simulink model "main_servo_laser"  (R2019b)
settings: Solver=VariableStepAuto  StartTime=0.0  StopTime=60  RelTol=1e-3
undefined symbols (not defined in the file): __PRM__SERIALIZED__DATA__, SubsystemReferenceBlock
settings Model: Creator=toons  LastModifiedBy=toons

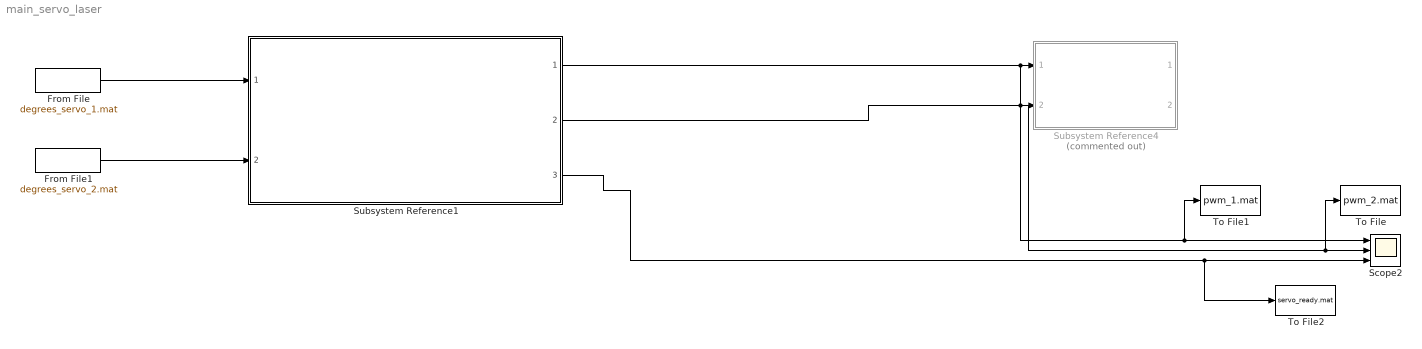
== system main_servo_laser ==
  From File : FromFile  FileName=degrees_servo_1.mat
  From File1 : FromFile  FileName=degrees_servo_2.mat
  Scope2 : Scope  NumInputPorts=3
  Subsystem Reference1 : Subsystem  BlockKeywords=__PRM__SERIALIZED__DATA__:SubsystemReferenceBlock  ReferencedSubsystem=MicroControllerPWM
  Subsystem Reference4 : Subsystem  Commented=on  BlockKeywords=__PRM__SERIALIZED__DATA__:SubsystemReferenceBlock  ReferencedSubsystem=ServoSimulation
  To File : ToFile  Filename=pwm_2.mat  SaveFormat=Timeseries
  To File1 : ToFile  Filename=pwm_1.mat  SaveFormat=Timeseries
  To File2 : ToFile  Filename=servo_ready.mat  SaveFormat=Timeseries
  wires:
  Subsystem Reference1/3 -> To File2/1, Scope2/3
  Subsystem Reference1/1 -> To File1/1, Scope2/1, Subsystem Reference4/1
  From File/1 -> Subsystem Reference1/1
  From File1/1 -> Subsystem Reference1/2
  Subsystem Reference1/2 -> To File/1, Scope2/2, Subsystem Reference4/2
